simulink model "flyback"  (R2021a)
settings: Solver=FixedStepDiscrete  StartTime=0.0  StopTime=0.020  FixedStep=Ts/1000  RelTol=1e-3
values from neighbouring files (symbols this model uses):
  C = 100e-6    (= 0.0001)    [flyback_filter.m]    (also in hw10_flyback_filter.m)
  Cb = n*Cf    [flyback_filter.m]    (also in hw10_flyback_filter.m = nf*Cf)
  Cf = 47e-6 * 3    (= 0.000141)    [flyback_filter.m]    (also in hw10_flyback_filter.m)
  D = 0.3    [flyback_filter.m]    (also in hw10_flyback_filter.m)
  L = 250e-6    (= 0.00025)    [flyback_filter.m]    (also in hw10_flyback_filter.m)
  Lf = ((1/(fo*2*pi))^2)/Cf    [flyback_filter.m]    (also in hw10_flyback_filter.m = 1/(ff^2)/4/pi/pi/Cf)
  N = 1/2    (= 0.5)    [flyback_filter.m]
  R = 5    [flyback_filter.m]    (also in hw10_flyback_filter.m)
  Rf = Rof*sqrt( ( (2+n) * (4+3*n) ) / ( (2*n^2) * (4+n) ) )    [flyback_filter.m]    (also in hw10_flyback_filter.m = Rof*sqrt( (2+nf)*(4+3*nf)/(2*nf^2*(4+nf)) ))
  Ts = 1/fsw    (= 5e-06)    [flyback_filter.m]    (also in hw10_flyback_filter.m)
  Vg = 48    [flyback_filter.m]    (also in hw10_flyback_filter.m)
libraries: spsSeriesRLCBranchLib x7, spsGroundLib x4, spsCurrentMeasurementLib x2, spsDCVoltageSourceLib x2, spsDiodeLib x2, spsIdealSwitchLib x2, spsLinearTransformerLib x2, spsPWMGeneratorDCDCLib x2, spsVoltageMeasurementLib x2, spspowerguiLib x1
settings Model: Creator=yoshi  LastModifiedBy=jneat

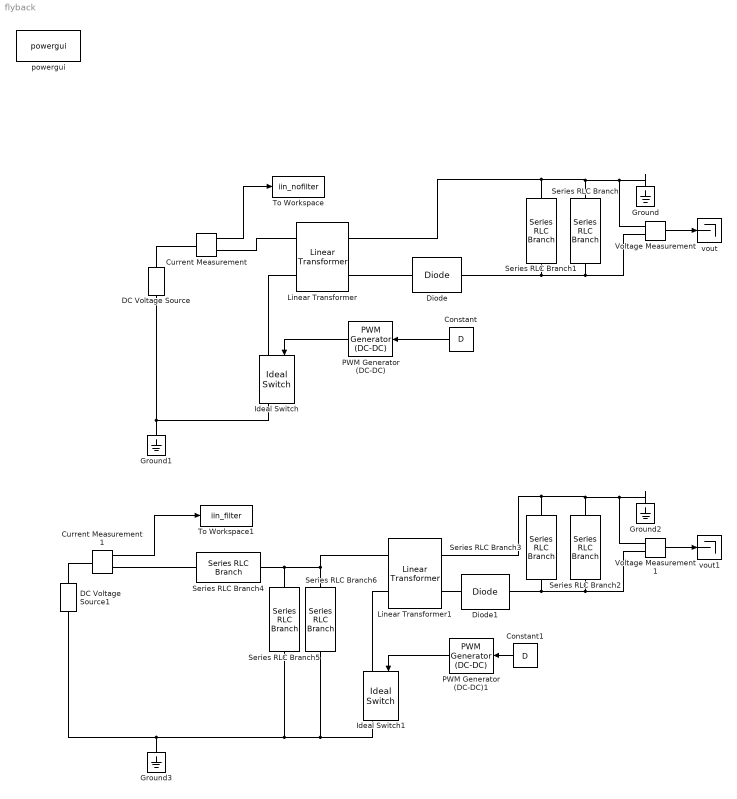
== system flyback ==
  Constant : Constant  Value=D
  Constant1 : Constant  Value=D
  Current Measurement : spsCurrentMeasurementLib/Current Measurement  PhasorSimulation=off  OutputType=Complex  PSBequivalent=0
  Current Measurement1 : spsCurrentMeasurementLib/Current Measurement  PhasorSimulation=off  OutputType=Complex  PSBequivalent=0
  DC Voltage Source : spsDCVoltageSourceLib/DC Voltage Source  Amplitude=Vg  Measurements=None
  DC Voltage Source1 : spsDCVoltageSourceLib/DC Voltage Source  Amplitude=Vg  Measurements=None
  Diode : spsDiodeLib/Diode  Ron=1e-6  Lon=0  Vf=0  IC=0  UseSnubber=0  Rs=500  Cs=0  Measurements=off
  Diode1 : spsDiodeLib/Diode  Ron=1e-6  Lon=0  Vf=0  IC=0  UseSnubber=0  Rs=500  Cs=0  Measurements=off
  Ground{,1..3} (4 alike) : spsGroundLib/Ground  LConnTagsString=a
  Ideal Switch : spsIdealSwitchLib/Ideal Switch  Ron=0.001  Lon=0  IC=0  Rs=1e5  Cs=inf  Measurements=on
  Ideal Switch1 : spsIdealSwitchLib/Ideal Switch  Ron=0.001  Lon=0  IC=0  Rs=1e5  Cs=inf  Measurements=on
  Linear Transformer : spsLinearTransformerLib/Linear Transformer  UNITS=SI  NominalPower=[ 250e6 60 ]  winding1=[7.35e5 0 0]  winding2=[N*7.35e5 0 0]  ThreeWindings=off  winding3=[3.15e+05 0.7938 0.084225]  RmLm=[1e6 L]  Measurements=Magnetization current  DataType=on
  Linear Transformer1 : spsLinearTransformerLib/Linear Transformer  UNITS=SI  NominalPower=[ 250e6 60 ]  winding1=[7.35e5 0 0]  winding2=[N*7.35e5 0 0]  ThreeWindings=off  winding3=[3.15e+05 0.7938 0.084225]  RmLm=[1e6 L]  Measurements=Magnetization current  DataType=on
  PWM Generator (DC-DC) : spsPWMGeneratorDCDCLib/PWM Generator (DC-DC)  Fsw=fsw  Ts=0
  PWM Generator (DC-DC)1 : spsPWMGeneratorDCDCLib/PWM Generator (DC-DC)  Fsw=fsw  Ts=0
  Series RLC Branch : spsSeriesRLCBranchLib/Series RLC Branch  LConnTagsString=__new0  RConnTagsString=__new0  BranchType=R  Resistance=R  Inductance=1e-3  SetiL0=off  InitialCurrent=0  Capacitance=1e-6  Setx0=off  InitialVoltage=0  Measurements=None
  Series RLC Branch1 : spsSeriesRLCBranchLib/Series RLC Branch  LConnTagsString=__new0  RConnTagsString=__new0  BranchType=C  Resistance=1  Inductance=1e-3  SetiL0=off  InitialCurrent=0  Capacitance=C  Setx0=off  InitialVoltage=0  Measurements=None
  Series RLC Branch2 : spsSeriesRLCBranchLib/Series RLC Branch  LConnTagsString=__new0  RConnTagsString=__new0  BranchType=R  Resistance=R  Inductance=1e-3  SetiL0=off  InitialCurrent=0  Capacitance=1e-6  Setx0=off  InitialVoltage=0  Measurements=None
  Series RLC Branch3 : spsSeriesRLCBranchLib/Series RLC Branch  LConnTagsString=__new0  RConnTagsString=__new0  BranchType=C  Resistance=1  Inductance=1e-3  SetiL0=off  InitialCurrent=0  Capacitance=C  Setx0=off  InitialVoltage=0  Measurements=None
  Series RLC Branch4 : spsSeriesRLCBranchLib/Series RLC Branch  LConnTagsString=__new0  RConnTagsString=__new0  BranchType=L  Resistance=1  Inductance=Lf  SetiL0=off  InitialCurrent=0  Capacitance=1e-6  Setx0=off  InitialVoltage=0  Measurements=None
  Series RLC Branch5 : spsSeriesRLCBranchLib/Series RLC Branch  LConnTagsString=__new0  RConnTagsString=__new0  BranchType=C  Resistance=1  Inductance=1e-3  SetiL0=off  InitialCurrent=0  Capacitance=Cf  Setx0=off  InitialVoltage=0  Measurements=None
  Series RLC Branch6 : spsSeriesRLCBranchLib/Series RLC Branch  LConnTagsString=__new0  RConnTagsString=__new0  BranchType=RC  Resistance=Rf  Inductance=1e-3  SetiL0=off  InitialCurrent=0  Capacitance=Cb  Setx0=off  InitialVoltage=0  Measurements=None
  To Workspace : ToWorkspace  VariableName=iin_nofilter  SampleTime=-1
  To Workspace1 : ToWorkspace  VariableName=iin_filter  SampleTime=-1
  Voltage Measurement : spsVoltageMeasurementLib/Voltage Measurement  PhasorSimulation=off  OutputType=Complex  PSBequivalent=0
  Voltage Measurement1 : spsVoltageMeasurementLib/Voltage Measurement  PhasorSimulation=off  OutputType=Complex  PSBequivalent=0
  powergui : spspowerguiLib/powergui  Priority=1  SimulationMode=Discrete  SampleTime=Ts/1000  frequency=60  Iterations=50  frequencyindice=0  Pbase=100e6  ErrMax=1e-4  UnitsV=kV  UnitsW=MW  buscounter=0  FunctionMessages=off  echomessages=off  EnableUseOfTLC=off  CurrentSourceSwitches=off  DisableSnubberDevices=off  DisableRonSwitches=off  DisableVfSwitches=off  DisplayEquations=off  AutomaticDiscreteSolvers=off  SolverType=Tustin/Backward Euler (TBE)  Interpol=off  ExternalGateDelay=off  methode=off  Ts=100  x0status=blocks  SPID=on  SwTol=0  HookPort=off  NonlinearTolerance=1e-4  nMaxIteration=100  ContinueOnMaxIteration=off  RestoreLinks=warning  ResistiveCurrentMeasurement=off  Frange=[0:2:500]  Ylog=off  Xlog=on  ShowGrid=off  save=off  variable=ZData  structure=0  ZoomFFT=off  StartTime=0.0  cycles=1  DisplayStyle=1  fundamental=60  FreqAxis=off  MaxFrequency=1000  frequencyindicesteady=1  RmsSteady=1  display=off
  vout : Terminator
  vout1 : Terminator
  wires:
  Voltage Measurement/1 -> vout/1
  PWM Generator (DC-DC)/1 -> Ideal Switch/1
  Constant/1 -> PWM Generator (DC-DC)/1
  Current Measurement/1 -> To Workspace/1
  Current Measurement1/1 -> To Workspace1/1
  Constant1/1 -> PWM Generator (DC-DC)1/1
  PWM Generator (DC-DC)1/1 -> Ideal Switch1/1
  Voltage Measurement1/1 -> vout1/1
  connections:
  Ideal Switch/LConn1 -- Linear Transformer/LConn2
  Ideal Switch/RConn1 -- Ground1/LConn1 -- DC Voltage Source/LConn1
  DC Voltage Source/RConn1 -- Current Measurement/LConn1
  Diode/RConn1 -- Voltage Measurement/LConn1 -- Series RLC Branch/RConn1 -- Series RLC Branch1/LConn1
  Series RLC Branch1/RConn1 -- Ground/LConn1 -- Voltage Measurement/LConn2 -- Series RLC Branch/LConn1 -- Linear Transformer/RConn1
  Diode/LConn1 -- Linear Transformer/RConn2
  Current Measurement/RConn1 -- Linear Transformer/LConn1
  Linear Transformer1/RConn1 -- Series RLC Branch3/RConn1 -- Ground2/LConn1 -- Voltage Measurement1/LConn2 -- Series RLC Branch2/LConn1
  Series RLC Branch3/LConn1 -- Diode1/RConn1 -- Voltage Measurement1/LConn1 -- Series RLC Branch2/RConn1
  DC Voltage Source1/LConn1 -- Series RLC Branch5/RConn1 -- Series RLC Branch6/RConn1 -- Ideal Switch1/RConn1 -- Ground3/LConn1
  DC Voltage Source1/RConn1 -- Current Measurement1/LConn1
  Ideal Switch1/LConn1 -- Linear Transformer1/LConn2
  Diode1/LConn1 -- Linear Transformer1/RConn2
  Series RLC Branch5/LConn1 -- Series RLC Branch6/LConn1 -- Linear Transformer1/LConn1 -- Series RLC Branch4/RConn1
  Series RLC Branch4/LConn1 -- Current Measurement1/RConn1
